simulink model "Mode_VOO"  (R2022b)
settings: Solver=FixedStepAuto  StartTime=0.0  StopTime=10.0  FixedStep=1e-3  RelTol=1e-3  EnableMultiTasking=on
undefined symbols (not defined in the file): D10, D11, D12, D2, D4, D5, D7, D8, D9, PTA0, PTA2, PTB23, PTB9, PTC3, PTC4, PTD0, PTD2, PTD3
libraries: frdmk64flib x10
settings Model: ExtModeTrigDuration=5  Creator=sarahalabdulrazzak  LastModifiedBy=kavem
settings SolverCC: AlgebraicLoopSolver=TrustRegion
settings OptimizationCC: EnhancedBackFolding=on  PassReuseOutputArgsAs=Individual arguments  ZeroExternalMemoryAtStartup=off  ZeroInternalMemoryAtStartup=off  MaxStackSize=64  OptimizeBlockOrder=speed  DifferentSizesBufferReuse=on  OptimizationCustomize=off  EfficientTunableParamExpr=on
settings DebuggingCC: ParameterTunabilityLossMsg=error  UnconnectedInputMsg=warning  UnconnectedOutputMsg=warning  UnconnectedLineMsg=warning  SFMachineParentedDataDiag=warning
settings HardwareCC: ProdBitPerPointer=32  ProdBitPerSizeT=32  ProdBitPerPtrDiffT=32  ProdLargestAtomicInteger=Long  ProdLargestAtomicFloat=Double  ProdWordSize=32  ProdHWDeviceType=ARM Compatible->ARM Cortex
settings ModelReferenceCC: EnableRefExpFcnMdlSchedulingChecks=on
settings SFSimCC: MATLABDynamicMemAlloc=off
settings RTWCC: Description=Embedded Coder  SystemTargetFile=ert.tlc  HardwareBoard=NXP FRDM-K64F  TLCOptions="-aInlineSetEventsForThisBaseRateFcn=TLC_FALSE -aSuppressMultiTaskScheduler=TLC_FALSE  -aRateBasedStepFcn=0"  TemplateMakefile=ert_default_tmf  Toolchain=GNU Tools for ARM Embedded Processors
settings CodeAppCC: ForceParamTrailComments=on  IgnoreCustomStorageClasses=off  OperatorAnnotations=on  SimulinkDataObjDesc=on  SFDataObjDesc=on  InsertBlockDesc=on

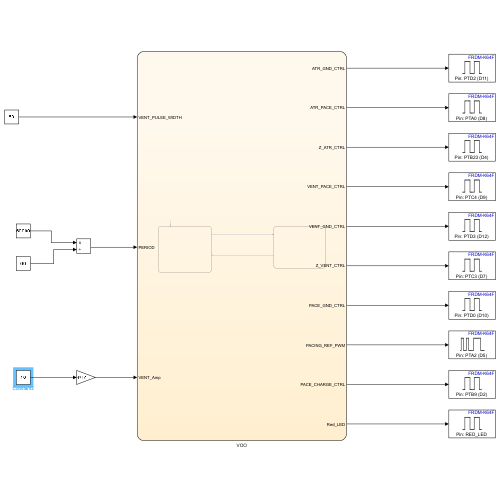
[thumbnail: Simulink's stored preview of the top-level diagram]
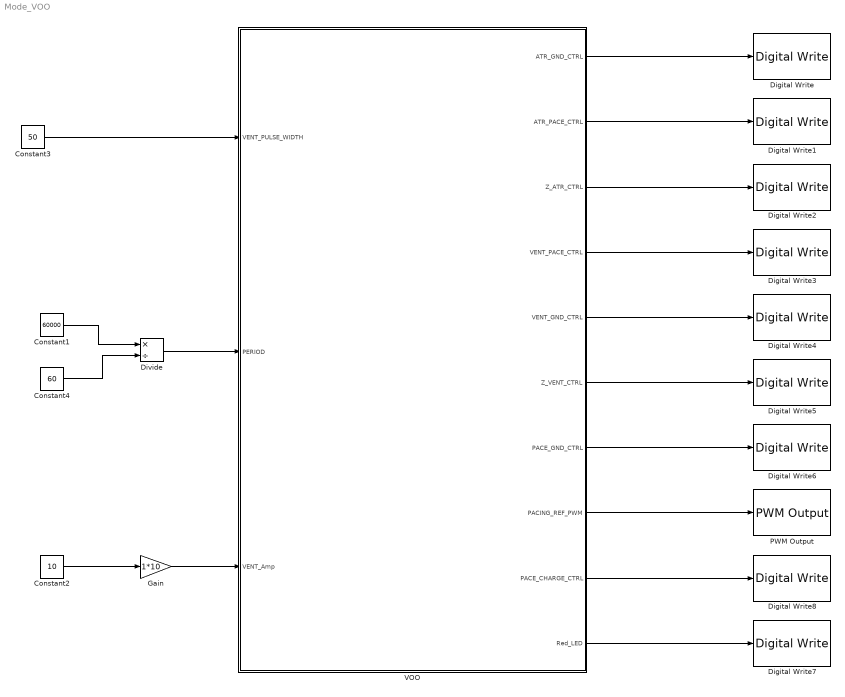
== system Mode_VOO ==
  Constant1 : Constant  Value=60000
  Constant2 : Constant  Value=10
  Constant3 : Constant  Value=50
  Constant4 : Constant  Value=60
  Digital Write : frdmk64flib/Digital Write  Whichpin=PTD2 (D11)
  Digital Write1 : frdmk64flib/Digital Write  Whichpin=PTA0 (D8)
  Digital Write2 : frdmk64flib/Digital Write  Whichpin=PTB23 (D4)
  Digital Write3 : frdmk64flib/Digital Write  Whichpin=PTC4 (D9)
  Digital Write4 : frdmk64flib/Digital Write  Whichpin=PTD3 (D12)
  Digital Write5 : frdmk64flib/Digital Write  Whichpin=PTC3 (D7)
  Digital Write6 : frdmk64flib/Digital Write  Whichpin=PTD0 (D10)
  Digital Write7 : frdmk64flib/Digital Write  Whichpin=RED_LED
  Digital Write8 : frdmk64flib/Digital Write  Whichpin=PTB9 (D2)
  Divide : Product  Inputs=*/
  Gain : Gain  Gain=1*10
  PWM Output : frdmk64flib/PWM Output  Whichpin=PTA2 (D5)  InitialFrequency=2000  InitialDutyCycle=0
  VOO : Stateflow chart  TreatAsAtomicUnit=on
  wires:
  VOO/1(ATR_GND_CTRL) -> Digital Write/1
  VOO/2(ATR_PACE_CTRL) -> Digital Write1/1
  VOO/3(Z_ATR_CTRL) -> Digital Write2/1
  VOO/4(VENT_PACE_CTRL) -> Digital Write3/1
  VOO/5(VENT_GND_CTRL) -> Digital Write4/1
  VOO/6(Z_VENT_CTRL) -> Digital Write5/1
  VOO/7(PACE_GND_CTRL) -> Digital Write6/1
  VOO/9(PACE_CHARGE_CTRL) -> Digital Write8/1
  Constant1/1 -> Divide/1
  Constant4/1 -> Divide/2
  Divide/1 -> VOO/2(PERIOD)
  VOO/10(Red_LED) -> Digital Write7/1
  VOO/8(PACING_REF_PWM) -> PWM Output/1
  Constant2/1 -> Gain/1
  Gain/1 -> VOO/3(VENT_Amp)
  Constant3/1 -> VOO/1(VENT_PULSE_WIDTH)

== stateflow chart Mode_VOO/VOO ==
  state CHARGING
    entry:
    %Charge primary capcitor C22
    ATR_PACE_CTRL=LOW
    VENT_PACE_CTRL=LOW
    PACING_REF_PWM = VENT_Amp
    PACE_CHARGE_CTRL = HIGH
    %Discharge block capacitor C21
    PACE_GND_CTRL = HIGH
    %VENT_PACE_CTRL = LOW
    Z_ATR_CTRL = LOW
    Z_VENT_CTRL = LOW
    %ATR_PACE_CTRL = LOW
    ATR_GND_CTRL = LOW
    VENT_GND_CTRL = HIGH
    %use LED  to verify state
    Red_LED=false
  state DISCHARGING
    entry:
    %Discharge C22 primary capacitor
    %Charge C21 block capacitor
    PACE_CHARGE_CTRL = LOW
    PACE_GND_CTRL = HIGH
    ATR_PACE_CTRL = LOW
    ATR_GND_CTRL = LOW
    Z_ATR_CTRL = LOW
    Z_VENT_CTRL = LOW
    VENT_GND_CTRL = LOW
    VENT_PACE_CTRL  = HIGH
    PACING_REF_PWM = VENT_Amp
    %use LED  to verify state
    Red_LED=true
  (default) -> CHARGING
  CHARGING -> DISCHARGING : [after(PERIOD - VENT_PULSE_WIDTH,msec)]
  DISCHARGING -> CHARGING : [after(VENT_PULSE_WIDTH,msec)]
  data: ATR_GND_CTRL output; ATR_PACE_CTRL output; Z_ATR_CTRL output; VENT_PACE_CTRL output; VENT_GND_CTRL output; Z_VENT_CTRL output; PACE_GND_CTRL output; PACING_REF_PWM output; PACE_CHARGE_CTRL output; VENT_PULSE_WIDTH input; PERIOD input; HIGH local =true; LOW local =false; VENT_Amp input; Red_LED output
